simulink model "test_ROS"  (R2018a)
settings: Solver=FixedStepDiscrete  StartTime=0.0  StopTime=inf  FixedStep=0.25  RelTol=1e-3
libraries: sldrtlib x1, robotlib x1
settings Model: Creator=silviobacci  LastModifiedBy=silviobacci

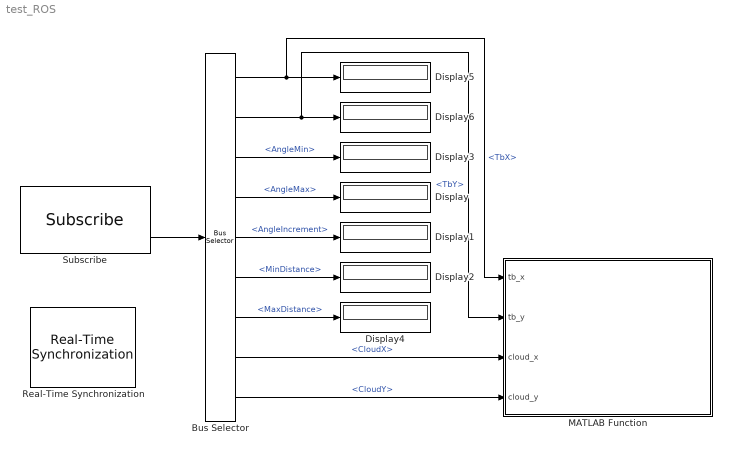
== system test_ROS ==
  Bus Selector : BusSelector  OutputSignals=TbX,TbY,AngleMin,AngleMax,AngleIncrement,MinDistance,MaxDistance,CloudX,CloudY
  Display{,1..6} (7 alike) : Display
  MATLAB Function : MATLAB Function  TreatAsAtomicUnit=on
  Real-Time Synchronization : sldrtlib/Real-Time Synchronization  SampleTime=0.25  MaxMissedTicks=10  ShowMissedTicks=off  YieldWhenWaiting=off
  Subscribe : robotlib/Subscribe  SourceLibraryInfo=This block requires Robotics System Toolbox  topicSource=Select from ROS network  topic=/env_constructor  messageType=turtlebot3_environment_scanner/tb_cloud_points  sampleTime=-1  messageQueueLength=1
      settings: SourceProductBaseCode=RO
  wires:
  Subscribe/2 -> Bus Selector/1
  Bus Selector/3 -> Display3/1  "<AngleMin>"
  Bus Selector/4 -> Display/1  "<AngleMax>"
  Bus Selector/5 -> Display1/1  "<AngleIncrement>"
  Bus Selector/6 -> Display2/1  "<MinDistance>"
  Bus Selector/7 -> Display4/1  "<MaxDistance>"
  Bus Selector/8 -> MATLAB Function/3(cloud_x)  "<CloudX>"
  Bus Selector/9 -> MATLAB Function/4(cloud_y)  "<CloudY>"
  Bus Selector/2 -> MATLAB Function/2(tb_y), Display6/1  "<TbY>"
  Bus Selector/1 -> MATLAB Function/1(tb_x), Display5/1  "<TbX>"

== matlab function test_ROS/MATLAB Function ==
  data: tb_x input; tb_y input; cloud_x input; cloud_y input
function plot_environment(tb_x, tb_y, cloud_x, cloud_y)

coder.extrinsic('scatter')
%plot(-tb_y, tb_x)
scatter(-cloud_y, cloud_x)
xlim([-3, 3])
ylim([-3, 3])
hold on
